simulink library "osqp_library"  (R2018b)
settings: Solver=VariableStepAuto  StartTime=0.0  StopTime=10.0  RelTol=1e-3
values from neighbouring files (symbols this model uses):
  A = block.DialogPrm(4).Data    [osqp_sfun.m]
  l = block.InputPort(8).Data    [osqp_sfun.m]
  m = block.DialogPrm(1).Data    [osqp_sfun.m]
  n = block.DialogPrm(2).Data    [osqp_sfun.m]
  P = block.DialogPrm(3).Data    [osqp_sfun.m]
  q = block.InputPort(7).Data    [osqp_sfun.m]
undefined symbols (not defined in the file or in its folder): osqp
settings Model: Creator=pgoulart  LastModifiedBy=pgoulart

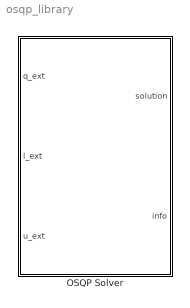
== system osqp_library ==
  OSQP Solver : Subsystem  mask{P=P, A=A, q=q, l=l, u=u, opts={'verbose',true}, refactor_style=Never, warmstart_style=Always, has_external_q_input=on, has_external_bound_input=on}
      mask prompts: opts "OSQP Settings"; refactor_style "Refactorisation"; warmstart_style "Warm starting"; has_external_q_input "External linear cost (q)"; has_external_bound_input "External bounds (l,u)"
      mask init:
      | osqp_block_init(gcb)
      mask TypeOptions refactor_style: Never | Always | Triggered
      mask TypeOptions warmstart_style: Never | Always | Triggered
      mask DialogControl ParameterGroupVar Prompt: OSQP Solver Data

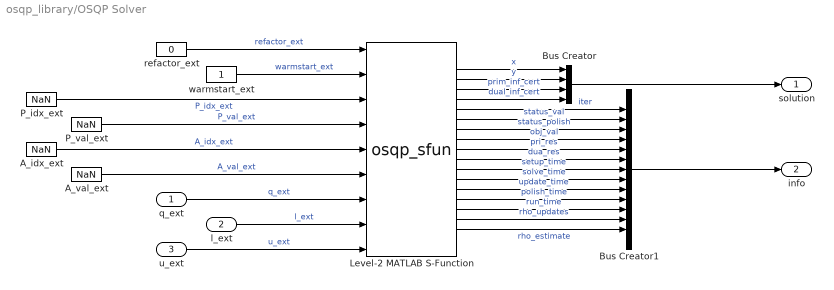
== system osqp_library/OSQP Solver ==
  q_ext : Inport
  l_ext : Inport  Port=2
  u_ext : Inport  Port=3
  A_idx_ext : Constant  Value=NaN
  A_val_ext : Constant  Value=NaN
  Bus Creator : BusCreator  Inputs=4
  Bus Creator1 : BusCreator  Inputs=13
  Level-2 MATLAB S-Function : M-S-Function  FunctionName=osqp_sfun  Parameters=m,n,P,A,q,l,u,osqp,opts
  P_idx_ext : Constant  Value=NaN
  P_val_ext : Constant  Value=NaN
  refactor_ext : Constant  Value=0
  warmstart_ext : Constant
  solution : Outport
  info : Outport  Port=2
  wires:
  warmstart_ext/1 -> Level-2 MATLAB S-Function/2  "warmstart_ext"
  l_ext/1 -> Level-2 MATLAB S-Function/8  "l_ext"
  A_idx_ext/1 -> Level-2 MATLAB S-Function/5  "A_idx_ext"
  P_idx_ext/1 -> Level-2 MATLAB S-Function/3  "P_idx_ext"
  Level-2 MATLAB S-Function/8 -> Bus Creator1/4  "obj_val"
  Level-2 MATLAB S-Function/15 -> Bus Creator1/11  "run_time"
  u_ext/1 -> Level-2 MATLAB S-Function/9  "u_ext"
  Level-2 MATLAB S-Function/9 -> Bus Creator1/5  "pri_res"
  Level-2 MATLAB S-Function/17 -> Bus Creator1/13  "rho_estimate"
  P_val_ext/1 -> Level-2 MATLAB S-Function/4  "P_val_ext"
  A_val_ext/1 -> Level-2 MATLAB S-Function/6  "A_val_ext"
  refactor_ext/1 -> Level-2 MATLAB S-Function/1  "refactor_ext"
  q_ext/1 -> Level-2 MATLAB S-Function/7  "q_ext"
  Level-2 MATLAB S-Function/12 -> Bus Creator1/8  "solve_time"
  Level-2 MATLAB S-Function/1 -> Bus Creator/1  "x"
  Level-2 MATLAB S-Function/4 -> Bus Creator/4  "dual_inf_cert"
  Level-2 MATLAB S-Function/2 -> Bus Creator/2  "y"
  Level-2 MATLAB S-Function/3 -> Bus Creator/3  "prim_inf_cert"
  Level-2 MATLAB S-Function/6 -> Bus Creator1/2  "status_val"
  Level-2 MATLAB S-Function/11 -> Bus Creator1/7  "setup_time"
  Level-2 MATLAB S-Function/14 -> Bus Creator1/10  "polish_time"
  Level-2 MATLAB S-Function/5 -> Bus Creator1/1  "iter"
  Level-2 MATLAB S-Function/7 -> Bus Creator1/3  "status_polish"
  Level-2 MATLAB S-Function/16 -> Bus Creator1/12  "rho_updates"
  Level-2 MATLAB S-Function/13 -> Bus Creator1/9  "update_time"
  Level-2 MATLAB S-Function/10 -> Bus Creator1/6  "dua_res"
  Bus Creator/1 -> solution/1
  Bus Creator1/1 -> info/1
